simulink model "fsk4_rx"  (R2020b)
settings: Solver=VariableStepAuto  StartTime=0.0  StopTime=2/100e3  RelTol=1e-3
PreLoadFcn:
  | setup_receiver
InitFcn:
  | setup_receiver;
  | fs=100e3;
undefined symbols (not defined in the file): AXI4, Lite
libraries: xbsIndex_r4 x242, hdlsllib x16, commrandsrc3 x2, dsphdlxfrm x1
(part 1 of 2)
settings Model: Creator=s1553558  LastModifiedBy=s1553558

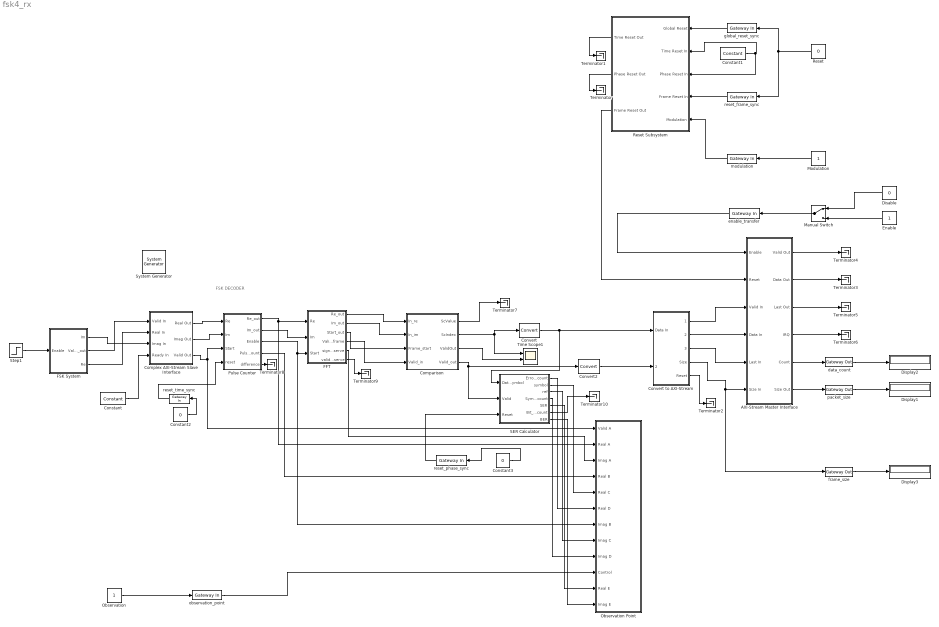
== system fsk4_rx ==
  note: FSK DECODER
  " System Generator" : xbsIndex_r4/ System Generator  Tag=genX  xilinxfamily=zynquplusRFSOC  part=xczu48dr  speed=-1-e  package=ffvg1517  synthesis_tool=Vivado  clock_wrapper=Clock Enables  directory=./netlist  proj_type=Vivado  Synth_file=Vivado Synthesis Defaults  Impl_file=Vivado Implementation Defaults  testbench=off  simulink_period=1/128e6  sysclk_period=(1/128e6)*1e9  dcm_input_clock_period=10  incr_netlist=off  trim_vbits=Everywhere in SubSystem  dbl_ovrd=According to Block Masks  core_generation=According to Block Masks  run_coregen=off  deprecated_control=off  eval_field=0  block_type=sysgen
  AXI-Stream Master Interface : Subsystem
  Comparison : Subsystem
  Complex AXI-Stream Slave Interface : Subsystem
  Constant : xbsIndex_r4/Constant  const=1.0  gui_display_data_type=Fixed-point  arith_type=Unsigned  n_bits=1  bin_pt=0  preci_type=Single  exp_width=8  frac_width=24  explicit_period=on  period=1/128e6  equ=P=C  opselect=C  inp2=PCIN>>17  opr=+  inp1=P  carry=CIN  dbl_ovrd=off  block_type=constant
  Constant1 : xbsIndex_r4/Constant  const=0  gui_display_data_type=Boolean  arith_type=Boolean  n_bits=16  bin_pt=14  preci_type=Single  exp_width=8  frac_width=24  explicit_period=on  period=1/128e6  equ=P=C  opselect=C  inp2=PCIN>>17  opr=+  inp1=P  carry=CIN  dbl_ovrd=off  block_type=constant
  Constant2 : Constant  Value=0
  Constant3 : Constant  Value=0
  Convert : xbsIndex_r4/Convert  gui_display_data_type=Fixed-point  arith_type=Unsigned  n_bits=8  bin_pt=0  float_type=Single  exp_bits=8  fraction_bits=24  quantization=Truncate  overflow=Wrap  en=off  latency=0  pipeline=off  dbl_ovrd=off  block_type=convert
  Convert to AXI-Stream : Subsystem
  Convert2 : xbsIndex_r4/Convert  gui_display_data_type=Boolean  arith_type=Boolean  n_bits=2  bin_pt=0  float_type=Single  exp_bits=8  fraction_bits=24  quantization=Truncate  overflow=Wrap  en=off  latency=0  pipeline=off  dbl_ovrd=off  block_type=convert
  Disable : Constant  Value=0  OutDataTypeStr=boolean  SampleTime=-1
  Display1 : Display
  Display2 : Display
  Display3 : Display
  Enable : Constant  OutDataTypeStr=boolean  SampleTime=-1
  FFT : Subsystem
  FSK System : Subsystem
  Manual Switch : ManualSwitch
  Modulation : Constant  OutDataTypeStr=boolean  SampleTime=-1
  Observation : Constant  OutDataTypeStr=uint32  SampleTime=-1
  Observation Point : Subsystem
  Pulse Counter : Subsystem
  Reset : Constant  Value=0  OutDataTypeStr=boolean  SampleTime=-1
  Reset Subsystem : Subsystem
  SER Calculator : Subsystem
  Step1 : Step  Time=32/128e6  SampleTime=32/128e6
  Terminator{,1..10} (11 alike) : Terminator
  Time Scope1 : Scope  NumInputPorts=2
  data_count : xbsIndex_r4/Gateway Out  inherit_from_input=on  hdl_port=on  rows=1  columns=1  UseAsDAC=off  DACChannel='1'  interface=AXI4-Lite  automatic_assignment=off  address_offset=32  intf_name=''  intf_description=''  timing_constraint=None  locs_specified=off  LOCs={}  io_standard={}  block_type=gatewayout
  enable_transfer : xbsIndex_r4/Gateway In  gui_display_data_type=Boolean  arith_type=Boolean  n_bits=16  bin_pt=14  preci_type=Single  exp_width=8  frac_width=24  rows=1  columns=1  quantization="Round  (unbiased: +/- Inf)"  overflow=Saturate  period=1/128e6  UseAsADC=off  ADCChannel='1'  interface=AXI4-Lite  automatic_assignment=off  address_offset=28  intf_name=''  intf_description=''  default_value=0  timing_constraint=None  locs_specified=off  LOCs={}  io_standard={}  inherit_from_input=off  hdl_port=on  dbl_ovrd=off  block_type=gatewayin
  frame_size : xbsIndex_r4/Gateway Out  inherit_from_input=on  hdl_port=on  rows=1  columns=1  UseAsDAC=off  DACChannel='1'  interface=AXI4-Lite  automatic_assignment=off  address_offset=16  intf_name=''  intf_description=''  timing_constraint=None  locs_specified=off  LOCs={}  io_standard={}  block_type=gatewayout
  global_reset_sync : xbsIndex_r4/Gateway In  gui_display_data_type=Boolean  arith_type=Boolean  n_bits=16  bin_pt=14  preci_type=Single  exp_width=8  frac_width=24  rows=1  columns=1  quantization="Round  (unbiased: +/- Inf)"  overflow=Saturate  period=1/4e6  UseAsADC=off  ADCChannel='1'  interface=AXI4-Lite  automatic_assignment=off  address_offset=56  intf_name=''  intf_description=''  default_value=1  timing_constraint=None  locs_specified=off  LOCs={}  io_standard={}  inherit_from_input=off  hdl_port=on  dbl_ovrd=off  block_type=gatewayin
  modulation : xbsIndex_r4/Gateway In  gui_display_data_type=Boolean  arith_type=Boolean  n_bits=16  bin_pt=14  preci_type=Single  exp_width=8  frac_width=24  rows=1  columns=1  quantization="Round  (unbiased: +/- Inf)"  overflow=Saturate  period=1/4e6  UseAsADC=off  ADCChannel='1'  interface=AXI4-Lite  automatic_assignment=off  address_offset=48  intf_name=''  intf_description=''  default_value=0  timing_constraint=None  locs_specified=off  LOCs={}  io_standard={}  inherit_from_input=off  hdl_port=on  dbl_ovrd=off  block_type=gatewayin
  observation_point : xbsIndex_r4/Gateway In  gui_display_data_type=Fixed-point  arith_type=Unsigned  n_bits=32  bin_pt=0  preci_type=Single  exp_width=8  frac_width=24  rows=1  columns=1  quantization="Round  (unbiased: +/- Inf)"  overflow=Saturate  period=1/128e6  UseAsADC=off  ADCChannel='1'  interface=AXI4-Lite  automatic_assignment=off  address_offset=36  intf_name=''  intf_description=''  default_value=0  timing_constraint=None  locs_specified=off  LOCs={}  io_standard={}  inherit_from_input=off  hdl_port=on  dbl_ovrd=off  block_type=gatewayin
  packet_size : xbsIndex_r4/Gateway Out  inherit_from_input=on  hdl_port=on  rows=1  columns=1  UseAsDAC=off  DACChannel='1'  interface=AXI4-Lite  automatic_assignment=off  address_offset=20  intf_name=''  intf_description=''  timing_constraint=None  locs_specified=off  LOCs={}  io_standard={}  block_type=gatewayout
  reset_frame_sync : xbsIndex_r4/Gateway In  gui_display_data_type=Boolean  arith_type=Boolean  n_bits=16  bin_pt=14  preci_type=Single  exp_width=8  frac_width=24  rows=1  columns=1  quantization="Round  (unbiased: +/- Inf)"  overflow=Saturate  period=1/4e6  UseAsADC=off  ADCChannel='1'  interface=AXI4-Lite  automatic_assignment=off  address_offset=8  intf_name=''  intf_description=''  default_value=1  timing_constraint=None  locs_specified=off  LOCs={}  io_standard={}  inherit_from_input=off  hdl_port=on  dbl_ovrd=off  block_type=gatewayin
  reset_phase_sync : xbsIndex_r4/Gateway In  gui_display_data_type=Boolean  arith_type=Boolean  n_bits=16  bin_pt=14  preci_type=Single  exp_width=8  frac_width=24  rows=1  columns=1  quantization="Round  (unbiased: +/- Inf)"  overflow=Saturate  period=1/4e6  UseAsADC=off  ADCChannel='1'  interface=AXI4-Lite  automatic_assignment=off  address_offset=4  intf_name=''  intf_description=''  default_value=1  timing_constraint=None  locs_specified=off  LOCs={}  io_standard={}  inherit_from_input=off  hdl_port=on  dbl_ovrd=off  block_type=gatewayin
  reset_time_sync : xbsIndex_r4/Gateway In  gui_display_data_type=Boolean  arith_type=Boolean  n_bits=16  bin_pt=14  preci_type=Single  exp_width=8  frac_width=24  rows=1  columns=1  quantization="Round  (unbiased: +/- Inf)"  overflow=Saturate  period=1/4e6  UseAsADC=off  ADCChannel='1'  interface=AXI4-Lite  automatic_assignment=off  address_offset=0  intf_name=''  intf_description=''  default_value=1  timing_constraint=None  locs_specified=off  LOCs={}  io_standard={}  inherit_from_input=off  hdl_port=on  dbl_ovrd=off  block_type=gatewayin
  wires:
  FSK System/3(Re) -> Complex AXI-Stream Slave Interface/2(Real In)
  FSK System/1(Im) -> Complex AXI-Stream Slave Interface/3(Imag In)
  FSK System/2(Valid_out) -> Complex AXI-Stream Slave Interface/1(Valid In)
  Step1/1 -> FSK System/1(Enable)
  Observation/1 -> observation_point/1
  Pulse Counter/3(Enable) -> Observation Point/7(Imag B), FFT/3(Start)
  FFT/2(Im_out) -> Comparison/2(In_im)
  FFT/1(Re_out) -> Comparison/1(In_re)
  Comparison/2(ScIndex) -> Time Scope1/1, Convert/1
  Pulse Counter/1(Re_out) -> Observation Point/2(Real A), FFT/1(Re)
  FFT/3(Start_out) -> Comparison/3(Frame_start)
  observation_point/1 -> Observation Point/10(Control)
  Pulse Counter/2(Im_out) -> FFT/2(Im)
  Constant1/1 -> Reset Subsystem/3(Phase Reset In), Reset Subsystem/2(Time Reset In)
  Modulation/1 -> modulation/1
  modulation/1 -> Reset Subsystem/5(Modulation)
  global_reset_sync/1 -> Reset Subsystem/1(Global Reset)
  reset_frame_sync/1 -> Reset Subsystem/4(Frame Reset In)
  Reset/1 -> global_reset_sync/1, reset_frame_sync/1
  Disable/1 -> Manual Switch/1
  enable_transfer/1 -> AXI-Stream Master Interface/1(Enable)
  Manual Switch/1 -> enable_transfer/1
  Enable/1 -> Manual Switch/2
  Reset Subsystem/3(Frame Reset Out) -> AXI-Stream Master Interface/2(Reset)
  Reset Subsystem/2(Phase Reset Out) -> Terminator/1
  Reset Subsystem/1(Time Reset Out) -> Terminator1/1
  Convert to AXI-Stream/1(Valid Out) -> AXI-Stream Master Interface/3(Valid In)
  Convert to AXI-Stream/2(Data Out) -> AXI-Stream Master Interface/4(Data In)
  Convert to AXI-Stream/3(Last Out) -> AXI-Stream Master Interface/5(Last In)
  Convert to AXI-Stream/5(Reset) -> Terminator2/1
  Convert to AXI-Stream/4(Size) -> frame_size/1, AXI-Stream Master Interface/6(Size In)
  AXI-Stream Master Interface/3(Last Out) -> Terminator5/1
  AXI-Stream Master Interface/4(IRQ) -> Terminator6/1
  AXI-Stream Master Interface/2(Data Out) -> Terminator3/1
  AXI-Stream Master Interface/1(Valid Out) -> Terminator4/1
  frame_size/1 -> Display3/1
  packet_size/1 -> Display1/1
  data_count/1 -> Display2/1
  AXI-Stream Master Interface/5(Count) -> data_count/1
  AXI-Stream Master Interface/6(Size Out) -> packet_size/1
  Complex AXI-Stream Slave Interface/2(Imag Out) -> Pulse Counter/2(Im)
  Complex AXI-Stream Slave Interface/1(Real Out) -> Pulse Counter/1(Re)
  Constant/1 -> Complex AXI-Stream Slave Interface/4(Ready In)
  Comparison/1(ScValue) -> Terminator7/1
  Complex AXI-Stream Slave Interface/3(Valid Out) -> Pulse Counter/3(Start), Observation Point/1(Valid A)
  FFT/4(Valid_frame) -> Comparison/4(Valid_in)
  Pulse Counter/4(Pulse Count) -> Observation Point/4(Real B)
  Comparison/4(Valid_out) -> Convert2/1, SER Calculator/2(Valid)
  Pulse Counter/5(difference) -> Terminator8/1
  reset_time_sync/1 -> Pulse Counter/4(reset)
  Constant2/1 -> reset_time_sync/1
  SER Calculator/2(symbol) -> Observation Point/5(Real C)
  SER Calculator/3(ref) -> Observation Point/8(Imag C)
  reset_phase_sync/1 -> SER Calculator/3(Reset)
  Constant3/1 -> reset_phase_sync/1
  Comparison/3(ValidOut) -> Time Scope1/2
  Convert/1 -> Convert to AXI-Stream/1(Data In), SER Calculator/1(Data_Symbol)
  Convert2/1 -> Convert to AXI-Stream/2(Valid In)
  FFT/5(signal_observe) -> Observation Point/3(Imag A)
  SER Calculator/4(Symbol_count) -> Observation Point/9(Imag D)
  FFT/6(valid_observe) -> Terminator9/1
  SER Calculator/7(BER) -> Observation Point/12(Imag E)
  SER Calculator/6(Bit_error_count) -> Terminator10/1
  SER Calculator/1(Error_count) -> Observation Point/6(Real D)
  SER Calculator/5(SER) -> Observation Point/11(Real E)

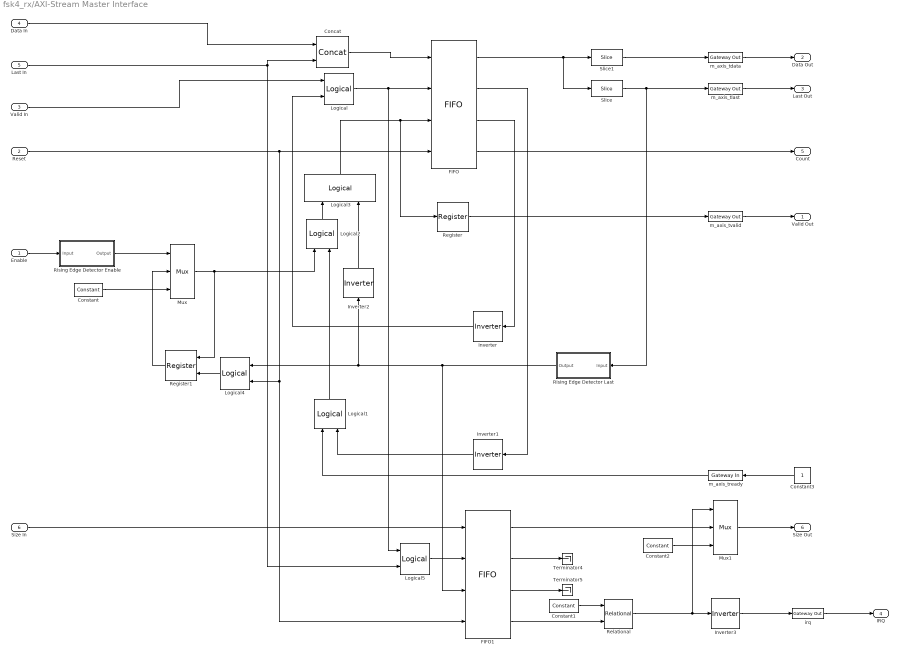
== system fsk4_rx/AXI-Stream Master Interface ==
  Enable : Inport
  Reset : Inport  Port=2
  Valid In : Inport  Port=3
  Data In : Inport  Port=4
  Last In : Inport  Port=5
  Size In : Inport  Port=6
  Concat : xbsIndex_r4/Concat  num_inputs=2  dbl_ovrd=off  block_type=concat
  Constant : xbsIndex_r4/Constant  const=1.0  gui_display_data_type=Boolean  arith_type=Boolean  n_bits=16  bin_pt=14  preci_type=Single  exp_width=8  frac_width=24  explicit_period=off  period=1  equ=P=C  opselect=C  inp2=PCIN>>17  opr=+  inp1=P  carry=CIN  dbl_ovrd=off  block_type=constant
  Constant1 : xbsIndex_r4/Constant  const=0  gui_display_data_type=Fixed-point  arith_type=Unsigned  n_bits=1  bin_pt=0  preci_type=Single  exp_width=8  frac_width=24  explicit_period=off  period=1  equ=P=C  opselect=C  inp2=PCIN>>17  opr=+  inp1=P  carry=CIN  dbl_ovrd=off  block_type=constant
  Constant2 : xbsIndex_r4/Constant  const=0  gui_display_data_type=Fixed-point  arith_type=Unsigned  n_bits=8  bin_pt=0  preci_type=Single  exp_width=8  frac_width=24  explicit_period=off  period=1  equ=P=C  opselect=C  inp2=PCIN>>17  opr=+  inp1=P  carry=CIN  dbl_ovrd=off  block_type=constant
  Constant3 : Constant  SampleTime=1/64e6
  FIFO : xbsIndex_r4/FIFO  mem_type=Block RAM  performance_options=Standard_FIFO  embedded_registers=off  depth=4K  percent_nbits=1  rst=on  rst_latency=2  en=off  use_dcount=on  use_percent_full_port=off  use_almost_empty=off  almost_empty_thresh=2  use_almost_full=off  use_rd_rst_busy=off  use_wr_rst_busy=off  almost_full_thresh=14  explicit_period=off  dbl_ovrd=off  simulation_type=fast_sim  block_type=fifo
  FIFO1 : xbsIndex_r4/FIFO  mem_type=Block RAM  performance_options=First_Word_Fall_Through  embedded_registers=off  depth=4K  percent_nbits=1  rst=on  rst_latency=2  en=off  use_dcount=on  use_percent_full_port=off  use_almost_empty=off  almost_empty_thresh=2  use_almost_full=off  use_rd_rst_busy=off  use_wr_rst_busy=off  almost_full_thresh=14  explicit_period=off  dbl_ovrd=off  simulation_type=fast_sim  block_type=fifo
  Inverter{,1..3} (4 alike) : xbsIndex_r4/Inverter  en=off  latency=0  dbl_ovrd=off  block_type=inv
  Logical{,1..3,5} (5 alike) : xbsIndex_r4/Logical  logical_function=AND  inputs=2  en=off  latency=0  precision=Full  arith_type=Unsigned  n_bits=16  bin_pt=0  align_bp=on  dbl_ovrd=off  block_type=logical
  Logical4 : xbsIndex_r4/Logical  logical_function=OR  inputs=2  en=off  latency=0  precision=Full  arith_type=Unsigned  n_bits=16  bin_pt=0  align_bp=on  dbl_ovrd=off  block_type=logical
  Mux : xbsIndex_r4/Mux  inputs=2  en=off  latency=0  precision=Full  arith_type=Unsigned  n_bits=16  bin_pt=14  quantization=Truncate  overflow=Wrap  dbl_ovrd=off  block_type=mux
  Mux1 : xbsIndex_r4/Mux  inputs=2  en=off  latency=0  precision=Full  arith_type=Unsigned  n_bits=16  bin_pt=14  quantization=Truncate  overflow=Wrap  dbl_ovrd=off  block_type=mux
  Register : xbsIndex_r4/Register  init=0  rst=off  en=off  dbl_ovrd=off  block_type=register
  Register1 : xbsIndex_r4/Register  init=0  rst=on  en=off  dbl_ovrd=off  block_type=register
  Relational : xbsIndex_r4/Relational  mode=a=b  op_type=Bool  en=off  latency=0  dbl_ovrd=off  block_type=relational
  Rising Edge Detector Enable : Subsystem
  Rising Edge Detector Last : Subsystem
  Slice : xbsIndex_r4/Slice  nbits=1  boolean_output=on  mode=Two Bit Locations  bit1=0  base1=LSB of Input  bit0=0  base0=LSB of Input  dbl_ovrd=off  block_type=slice
  Slice1 : xbsIndex_r4/Slice  nbits=1  boolean_output=off  mode=Two Bit Locations  bit1=8  base1=LSB of Input  bit0=1  base0=LSB of Input  dbl_ovrd=off  block_type=slice
  Terminator4 : Terminator
  Terminator5 : Terminator
  irq : xbsIndex_r4/Gateway Out  inherit_from_input=on  hdl_port=on  rows=1  columns=1  UseAsDAC=off  DACChannel='1'  interface=Interrupt  automatic_assignment=off  address_offset=36  intf_name=''  intf_description=''  timing_constraint=None  locs_specified=off  LOCs={}  io_standard={}  block_type=gatewayout
  m_axis_tdata : xbsIndex_r4/Gateway Out  inherit_from_input=on  hdl_port=on  rows=1  columns=1  UseAsDAC=off  DACChannel='1'  interface=None  automatic_assignment=on  address_offset=hex2dec('00')  intf_name=''  intf_description=''  timing_constraint=None  locs_specified=off  LOCs={}  io_standard={}  block_type=gatewayout
  m_axis_tlast : xbsIndex_r4/Gateway Out  inherit_from_input=on  hdl_port=on  rows=1  columns=1  UseAsDAC=off  DACChannel='1'  interface=None  automatic_assignment=on  address_offset=hex2dec('00')  intf_name=''  intf_description=''  timing_constraint=None  locs_specified=off  LOCs={}  io_standard={}  block_type=gatewayout
  m_axis_tready : xbsIndex_r4/Gateway In  gui_display_data_type=Boolean  arith_type=Boolean  n_bits=16  bin_pt=14  preci_type=Single  exp_width=8  frac_width=24  rows=1  columns=1  quantization="Round  (unbiased: +/- Inf)"  overflow=Saturate  period=1/128e6  UseAsADC=off  ADCChannel='1'  interface=None  automatic_assignment=on  address_offset=hex2dec('00')  intf_name=''  intf_description=''  default_value=0  timing_constraint=None  locs_specified=off  LOCs={}  io_standard={}  inherit_from_input=off  hdl_port=on  dbl_ovrd=off  block_type=gatewayin
  m_axis_tvalid : xbsIndex_r4/Gateway Out  inherit_from_input=on  hdl_port=on  rows=1  columns=1  UseAsDAC=off  DACChannel='1'  interface=None  automatic_assignment=on  address_offset=hex2dec('00')  intf_name=''  intf_description=''  timing_constraint=None  locs_specified=off  LOCs={}  io_standard={}  block_type=gatewayout
  Valid Out : Outport  VectorParamsAs1DForOutWhenUnconnected=off
  Data Out : Outport  Port=2  VectorParamsAs1DForOutWhenUnconnected=off
  Last Out : Outport  Port=3  VectorParamsAs1DForOutWhenUnconnected=off
  IRQ : Outport  Port=4  VectorParamsAs1DForOutWhenUnconnected=off
  Count : Outport  Port=5  VectorParamsAs1DForOutWhenUnconnected=off
  Size Out : Outport  Port=6  VectorParamsAs1DForOutWhenUnconnected=off
  wires:
  irq/1 -> IRQ/1
  Constant3/1 -> m_axis_tready/1
  Size In/1 -> FIFO1/1
  m_axis_tvalid/1 -> Valid Out/1
  m_axis_tlast/1 -> Last Out/1
  m_axis_tdata/1 -> Data Out/1
  FIFO/1 -> Slice1/1, Slice/1
  Logical/1 -> Logical5/1, FIFO/2
  FIFO/3 -> Inverter/1
  Inverter/1 -> Logical/2
  FIFO/2 -> Inverter1/1
  Inverter1/1 -> Logical1/2
  m_axis_tready/1 -> Logical1/1
  Concat/1 -> FIFO/1
  FIFO/4 -> Count/1
  Slice1/1 -> m_axis_tdata/1
  Register/1 -> m_axis_tvalid/1
  Logical1/1 -> Logical2/2
  Mux/1 -> Register1/1, Logical2/1
  Rising Edge Detector Enable/1(Output) -> Mux/1
  Register1/1 -> Mux/2
  Constant/1 -> Mux/3
  Enable/1 -> Rising Edge Detector Enable/1(Input)
  Slice/1 -> Rising Edge Detector Last/1(Input), m_axis_tlast/1
  Rising Edge Detector Last/1(Output) -> FIFO1/3, Inverter2/1, Logical4/1
  Logical3/1 -> FIFO/3, Register/1
  Logical2/1 -> Logical3/1
  Inverter2/1 -> Logical3/2
  Logical4/1 -> Register1/2
  FIFO1/2 -> Terminator4/1
  FIFO1/3 -> Terminator5/1
  FIFO1/4 -> Relational/2
  Logical5/1 -> FIFO1/2
  Constant1/1 -> Relational/1
  FIFO1/1 -> Mux1/2
  Mux1/1 -> Size Out/1
  Relational/1 -> Inverter3/1, Mux1/1
  Constant2/1 -> Mux1/3
  Inverter3/1 -> irq/1
  Data In/1 -> Concat/1
  Last In/1 -> Logical5/2, Concat/2
  Valid In/1 -> Logical/1
  Reset/1 -> FIFO/4, Logical4/2, FIFO1/4

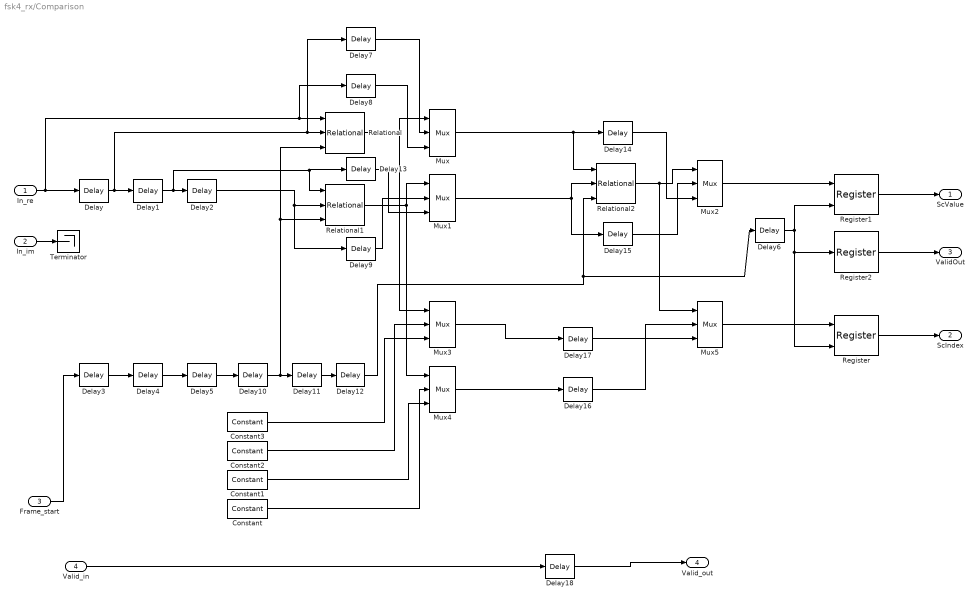
== system fsk4_rx/Comparison ==
  In_re : Inport
  In_im : Inport  Port=2
  Frame_start : Inport  Port=3
  Valid_in : Inport  Port=4
  Constant : xbsIndex_r4/Constant  const=0  gui_display_data_type=Fixed-point  arith_type=Unsigned  n_bits=16  bin_pt=14  preci_type=Single  exp_width=8  frac_width=24  explicit_period=on  period=1/128e6  equ=P=C  opselect=C  inp2=PCIN>>17  opr=+  inp1=P  carry=CIN  dbl_ovrd=off  block_type=constant
  Constant1 : xbsIndex_r4/Constant  const=1  gui_display_data_type=Fixed-point  arith_type=Unsigned  n_bits=16  bin_pt=14  preci_type=Single  exp_width=8  frac_width=24  explicit_period=on  period=1/128e6  equ=P=C  opselect=C  inp2=PCIN>>17  opr=+  inp1=P  carry=CIN  dbl_ovrd=off  block_type=constant
  Constant2 : xbsIndex_r4/Constant  const=2.0  gui_display_data_type=Fixed-point  arith_type=Unsigned  n_bits=16  bin_pt=14  preci_type=Single  exp_width=8  frac_width=24  explicit_period=on  period=1/128e6  equ=P=C  opselect=C  inp2=PCIN>>17  opr=+  inp1=P  carry=CIN  dbl_ovrd=off  block_type=constant
  Constant3 : xbsIndex_r4/Constant  const=3  gui_display_data_type=Fixed-point  arith_type=Unsigned  n_bits=16  bin_pt=14  preci_type=Single  exp_width=8  frac_width=24  explicit_period=on  period=1/128e6  equ=P=C  opselect=C  inp2=PCIN>>17  opr=+  inp1=P  carry=CIN  dbl_ovrd=off  block_type=constant
  Delay{,1..5,7..17} (17 alike) : xbsIndex_r4/Delay  rst=off  infoeditControl=Selection of Reset will increase slice count due to use of real FFs and instead of SRLs  en=off  latency=1  reg_retiming=off  dbl_ovrd=off  block_type=delay
  Delay18 : xbsIndex_r4/Delay  rst=off  infoeditControl=Selection of Reset will increase slice count due to use of real FFs and instead of SRLs  en=off  latency=8  reg_retiming=off  dbl_ovrd=off  block_type=delay
  Delay6 : xbsIndex_r4/Delay  rst=off  infoeditControl=Selection of Reset will increase slice count due to use of real FFs and instead of SRLs  en=off  latency=2  reg_retiming=off  dbl_ovrd=off  block_type=delay
  Mux{,1,3..4} (4 alike) : xbsIndex_r4/Mux  inputs=2  en=off  latency=1  precision=Full  arith_type=Unsigned  n_bits=16  bin_pt=14  quantization=Truncate  overflow=Wrap  dbl_ovrd=off  block_type=mux
  Mux2 : xbsIndex_r4/Mux  inputs=2  en=off  latency=1  precision=Full  arith_type="Signed  (2's comp)"  n_bits=16  bin_pt=14  quantization=Truncate  overflow=Wrap  dbl_ovrd=off  block_type=mux
  Mux5 : xbsIndex_r4/Mux  inputs=2  en=off  latency=1  precision=Full  arith_type="Signed  (2's comp)"  n_bits=16  bin_pt=14  quantization=Truncate  overflow=Wrap  dbl_ovrd=off  block_type=mux
  Register : xbsIndex_r4/Register  init=0  rst=off  en=on  dbl_ovrd=off  block_type=register
  Register1 : xbsIndex_r4/Register  init=0  rst=off  en=on  dbl_ovrd=off  block_type=register
  Register2 : xbsIndex_r4/Register  init=0  rst=off  en=off  dbl_ovrd=off  block_type=register
  Relational : xbsIndex_r4/Relational  mode=a>=b  op_type=Bool  en=on  latency=1  dbl_ovrd=off  block_type=relational
  Relational1 : xbsIndex_r4/Relational  mode=a>=b  op_type=Bool  en=on  latency=1  dbl_ovrd=off  block_type=relational
  Relational2 : xbsIndex_r4/Relational  mode=a>=b  op_type=Bool  en=on  latency=1  dbl_ovrd=off  block_type=relational
  Terminator : Terminator
  ScValue : Outport
  ScIndex : Outport  Port=2
  ValidOut : Outport  Port=3
  Valid_out : Outport  Port=4
  wires:
  Frame_start/1 -> Delay3/1
  Register1/1 -> ScValue/1
  In_re/1 -> Delay/1, Delay8/1, Relational/1
  Delay/1 -> Delay1/1, Delay7/1, Relational/2
  Delay2/1 -> Relational1/2, Delay9/1
  Relational/1 -> Mux/1, Mux3/1
  Mux/1 -> Relational2/1, Delay14/1
  Relational1/1 -> Mux4/1, Mux1/1
  Mux1/1 -> Delay15/1, Relational2/2
  Relational2/1 -> Mux5/1, Mux2/1
  Mux3/1 -> Delay17/1
  Mux4/1 -> Delay16/1
  Mux5/1 -> Register/1
  Register/1 -> ScIndex/1
  Delay10/1 -> Relational1/3, Relational/3, Delay11/1
  Delay3/1 -> Delay4/1
  Delay4/1 -> Delay5/1
  Delay5/1 -> Delay10/1
  Delay1/1 -> Relational1/1, Delay13/1, Delay2/1
  Delay11/1 -> Delay12/1
  Delay6/1 -> Register2/1, Register/2, Register1/2
  In_im/1 -> Terminator/1
  Delay7/1 -> Mux/2
  Delay8/1 -> Mux/3
  Delay9/1 -> Mux1/2
  Delay13/1 -> Mux1/3
  Delay14/1 -> Mux2/3
  Delay15/1 -> Mux2/2
  Mux2/1 -> Register1/1
  Delay12/1 -> Relational2/3, Delay6/1
  Constant3/1 -> Mux3/3
  Constant2/1 -> Mux3/2
  Constant/1 -> Mux4/2
  Constant1/1 -> Mux4/3
  Delay16/1 -> Mux5/2
  Delay17/1 -> Mux5/3
  Register2/1 -> ValidOut/1
  Valid_in/1 -> Delay18/1
  Delay18/1 -> Valid_out/1

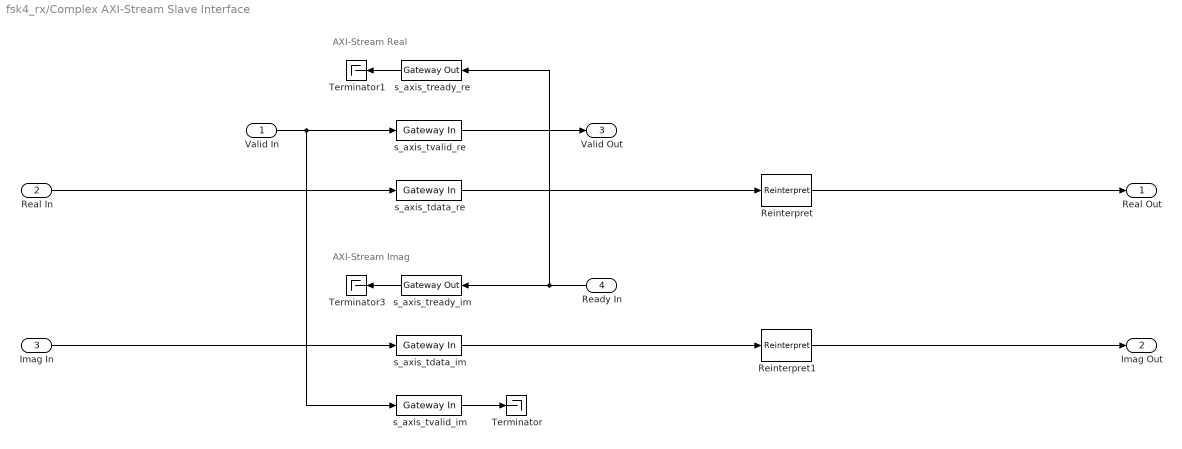
== system fsk4_rx/Complex AXI-Stream Slave Interface ==
  note: AXI-Stream Real
  note: AXI-Stream Imag
  Valid In : Inport
  Real In : Inport  Port=2
  Imag In : Inport  Port=3
  Ready In : Inport  Port=4
  Reinterpret : xbsIndex_r4/Reinterpret  force_arith_type=on  arith_type="Signed  (2's comp)"  force_bin_pt=on  bin_pt=14  block_type=reinterpret
  Reinterpret1 : xbsIndex_r4/Reinterpret  force_arith_type=on  arith_type="Signed  (2's comp)"  force_bin_pt=on  bin_pt=14  block_type=reinterpret
  Terminator : Terminator
  Terminator1 : Terminator
  Terminator3 : Terminator
  s_axis_tdata_im : xbsIndex_r4/Gateway In  gui_display_data_type=Fixed-point  arith_type=Unsigned  n_bits=16  bin_pt=0  preci_type=Double  exp_width=8  frac_width=24  rows=1  columns=1  quantization="Round  (unbiased: +/- Inf)"  overflow=Saturate  period=1/128e6  UseAsADC=off  ADCChannel='1'  interface=None  automatic_assignment=on  address_offset=hex2dec('00')  intf_name=''  intf_description=''  default_value=0  timing_constraint=None  locs_specified=off  LOCs={}  io_standard={}  inherit_from_input=off  hdl_port=on  dbl_ovrd=off  block_type=gatewayin
  s_axis_tdata_re : xbsIndex_r4/Gateway In  gui_display_data_type=Fixed-point  arith_type=Unsigned  n_bits=16  bin_pt=0  preci_type=Double  exp_width=8  frac_width=24  rows=1  columns=1  quantization="Round  (unbiased: +/- Inf)"  overflow=Saturate  period=1/128e6  UseAsADC=off  ADCChannel='1'  interface=None  automatic_assignment=on  address_offset=hex2dec('00')  intf_name=''  intf_description=''  default_value=0  timing_constraint=None  locs_specified=off  LOCs={}  io_standard={}  inherit_from_input=off  hdl_port=on  dbl_ovrd=off  block_type=gatewayin
  s_axis_tready_im : xbsIndex_r4/Gateway Out  inherit_from_input=off  hdl_port=on  rows=1  columns=1  UseAsDAC=off  DACChannel='1'  interface=None  automatic_assignment=on  address_offset=hex2dec('00')  intf_name=''  intf_description=''  timing_constraint=None  locs_specified=off  LOCs={}  io_standard={}  block_type=gatewayout
  s_axis_tready_re : xbsIndex_r4/Gateway Out  inherit_from_input=off  hdl_port=on  rows=1  columns=1  UseAsDAC=off  DACChannel='1'  interface=None  automatic_assignment=on  address_offset=hex2dec('00')  intf_name=''  intf_description=''  timing_constraint=None  locs_specified=off  LOCs={}  io_standard={}  block_type=gatewayout
  s_axis_tvalid_im : xbsIndex_r4/Gateway In  gui_display_data_type=Boolean  arith_type=Boolean  n_bits=16  bin_pt=14  preci_type=Single  exp_width=8  frac_width=24  rows=1  columns=1  quantization="Round  (unbiased: +/- Inf)"  overflow=Saturate  period=1/128e6  UseAsADC=off  ADCChannel='1'  interface=None  automatic_assignment=on  address_offset=hex2dec('00')  intf_name=''  intf_description=''  default_value=0  timing_constraint=None  locs_specified=off  LOCs={}  io_standard={}  inherit_from_input=off  hdl_port=on  dbl_ovrd=off  block_type=gatewayin
  s_axis_tvalid_re : xbsIndex_r4/Gateway In  gui_display_data_type=Boolean  arith_type=Boolean  n_bits=32  bin_pt=0  preci_type=Single  exp_width=8  frac_width=24  rows=1  columns=1  quantization="Round  (unbiased: +/- Inf)"  overflow=Saturate  period=1/128e6  UseAsADC=off  ADCChannel='1'  interface=None  automatic_assignment=on  address_offset=hex2dec('00')  intf_name=''  intf_description=''  default_value=0  timing_constraint=None  locs_specified=off  LOCs={}  io_standard={}  inherit_from_input=off  hdl_port=on  dbl_ovrd=off  block_type=gatewayin
  Real Out : Outport  VectorParamsAs1DForOutWhenUnconnected=off
  Imag Out : Outport  Port=2  VectorParamsAs1DForOutWhenUnconnected=off
  Valid Out : Outport  Port=3  VectorParamsAs1DForOutWhenUnconnected=off
  wires:
  s_axis_tready_re/1 -> Terminator1/1
  Valid In/1 -> s_axis_tvalid_re/1, s_axis_tvalid_im/1
  Ready In/1 -> s_axis_tready_im/1, s_axis_tready_re/1
  s_axis_tvalid_re/1 -> Valid Out/1
  s_axis_tvalid_im/1 -> Terminator/1
  s_axis_tready_im/1 -> Terminator3/1
  Imag In/1 -> s_axis_tdata_im/1
  Real In/1 -> s_axis_tdata_re/1
  s_axis_tdata_re/1 -> Reinterpret/1
  Reinterpret1/1 -> Imag Out/1
  s_axis_tdata_im/1 -> Reinterpret1/1
  Reinterpret/1 -> Real Out/1

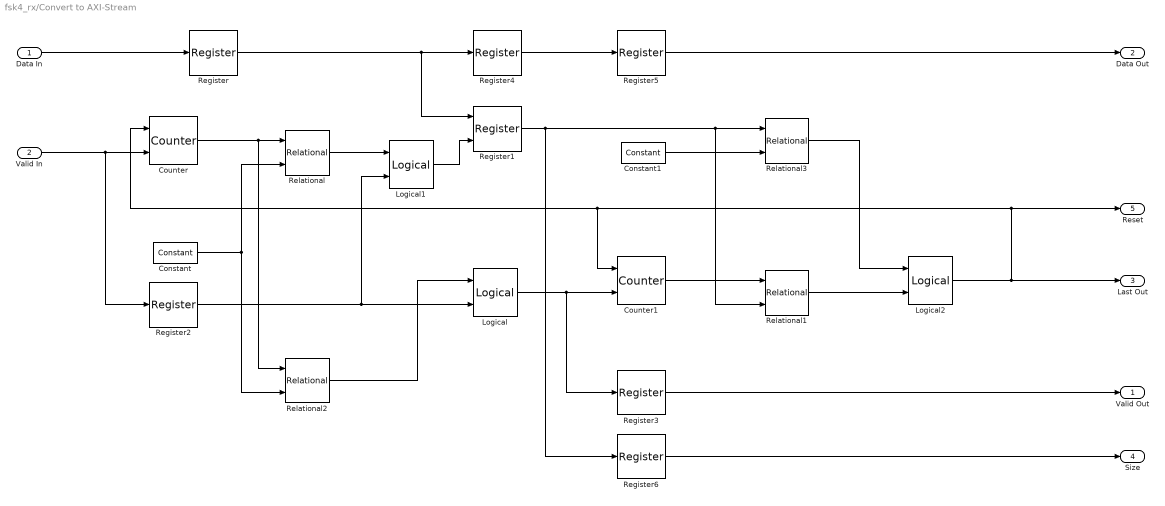
== system fsk4_rx/Convert to AXI-Stream ==
  Data In : Inport
  Valid In : Inport  Port=2
  Constant : xbsIndex_r4/Constant  const=1.0  gui_display_data_type=Fixed-point  arith_type=Unsigned  n_bits=1  bin_pt=0  preci_type=Single  exp_width=8  frac_width=24  explicit_period=off  period=1  equ=P=C  opselect=C  inp2=PCIN>>17  opr=+  inp1=P  carry=CIN  dbl_ovrd=off  block_type=constant
  Constant1 : xbsIndex_r4/Constant  const=0  gui_display_data_type=Fixed-point  arith_type=Unsigned  n_bits=1  bin_pt=0  preci_type=Single  exp_width=8  frac_width=24  explicit_period=off  period=1  equ=P=C  opselect=C  inp2=PCIN>>17  opr=+  inp1=P  carry=CIN  dbl_ovrd=off  block_type=constant
  Counter : xbsIndex_r4/Counter  cnt_type=Free Running  cnt_to=Inf  operation=Up  start_count=0  cnt_by_val=1  arith_type=Unsigned  n_bits=32  bin_pt=0  load_pin=off  rst=on  en=on  explicit_period=off  period=1  use_behavioral_HDL=off  implementation=Fabric  dbl_ovrd=off  block_type=counter
  Counter1 : xbsIndex_r4/Counter  cnt_type=Free Running  cnt_to=Inf  operation=Up  start_count=0  cnt_by_val=1  arith_type=Unsigned  n_bits=32  bin_pt=0  load_pin=off  rst=on  en=on  explicit_period=off  period=1  use_behavioral_HDL=off  implementation=Fabric  dbl_ovrd=off  block_type=counter
  Logical : xbsIndex_r4/Logical  logical_function=AND  inputs=2  en=off  latency=1  precision=Full  arith_type=Unsigned  n_bits=16  bin_pt=0  align_bp=on  dbl_ovrd=off  block_type=logical
  Logical1 : xbsIndex_r4/Logical  logical_function=AND  inputs=2  en=off  latency=0  precision=Full  arith_type=Unsigned  n_bits=16  bin_pt=0  align_bp=on  dbl_ovrd=off  block_type=logical
  Logical2 : xbsIndex_r4/Logical  logical_function=AND  inputs=2  en=off  latency=0  precision=Full  arith_type=Unsigned  n_bits=16  bin_pt=0  align_bp=on  dbl_ovrd=off  block_type=logical
  Register{,2..6} (6 alike) : xbsIndex_r4/Register  init=0  rst=off  en=off  dbl_ovrd=off  block_type=register
  Register1 : xbsIndex_r4/Register  init=0  rst=off  en=on  dbl_ovrd=off  block_type=register
  Relational : xbsIndex_r4/Relational  mode=a=b  op_type=Bool  en=off  latency=0  dbl_ovrd=off  block_type=relational
  Relational1 : xbsIndex_r4/Relational  mode=a>=b  op_type=Bool  en=off  latency=0  dbl_ovrd=off  block_type=relational
  Relational2 : xbsIndex_r4/Relational  mode=a>b  op_type=Bool  en=off  latency=0  dbl_ovrd=off  block_type=relational
  Relational3 : xbsIndex_r4/Relational  mode=a!=b  op_type=Bool  en=off  latency=0  dbl_ovrd=off  block_type=relational
  Valid Out : Outport  VectorParamsAs1DForOutWhenUnconnected=off
  Data Out : Outport  Port=2  VectorParamsAs1DForOutWhenUnconnected=off
  Last Out : Outport  Port=3  VectorParamsAs1DForOutWhenUnconnected=off
  Size : Outport  Port=4  VectorParamsAs1DForOutWhenUnconnected=off
  Reset : Outport  Port=5  VectorParamsAs1DForOutWhenUnconnected=off
  wires:
  Valid In/1 -> Register2/1, Counter/2
  Counter/1 -> Relational2/1, Relational/1
  Data In/1 -> Register/1
  Register/1 -> Register4/1, Register1/1
  Logical/1 -> Register3/1, Counter1/2
  Counter1/1 -> Relational1/1
  Register1/1 -> Register6/1, Relational3/1, Relational1/2
  Register2/1 -> Logical1/2, Logical/2
  Register3/1 -> Valid Out/1
  Register4/1 -> Register5/1
  Register5/1 -> Data Out/1
  Constant/1 -> Relational/2, Relational2/2
  Relational2/1 -> Logical/1
  Relational/1 -> Logical1/1
  Logical1/1 -> Register1/2
  Constant1/1 -> Relational3/2
  Relational3/1 -> Logical2/1
  Relational1/1 -> Logical2/2
  Logical2/1 -> Counter/1, Counter1/1, Reset/1, Last Out/1
  Register6/1 -> Size/1

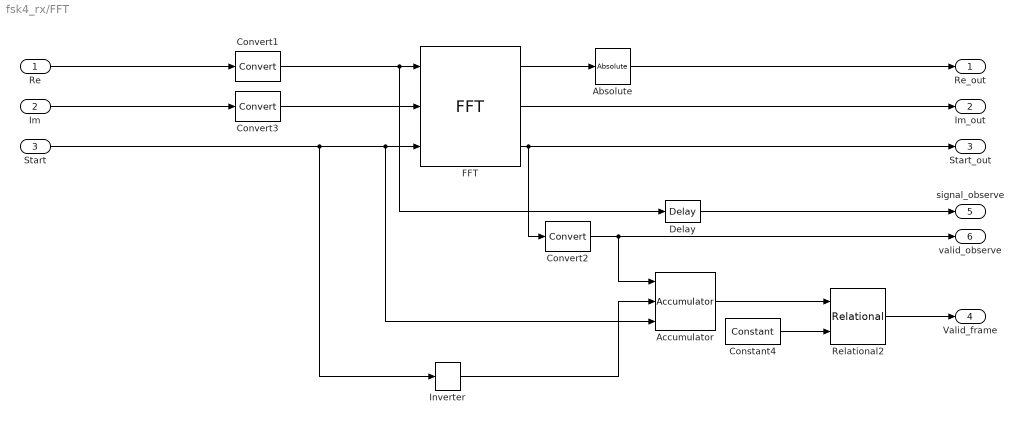
== system fsk4_rx/FFT ==
  Re : Inport
  Im : Inport  Port=2
  Start : Inport  Port=3
  Absolute : xbsIndex_r4/Absolute  precision=Full  arith_type=Unsigned  n_bits=16  bin_pt=14  quantization=Truncate  overflow=Wrap  en=off  latency=0  dbl_ovrd=off  block_type=abs
  Accumulator : xbsIndex_r4/Accumulator  operation=Add  n_bits=54  overflow=Wrap  scale=1  rst=on  hasbypass=off  infoeditControl=reset for floating point data type must be asserted for a minimum of 2 cycles  en=on  latency=0  msb_inp=100  msb=100  lsb=-100  use_behavioral_HDL=on  implementation=Fabric  dbl_ovrd=off  block_type=accum
  Constant4 : xbsIndex_r4/Constant  const=0.1  gui_display_data_type=Fixed-point  arith_type=Unsigned  n_bits=16  bin_pt=14  preci_type=Single  exp_width=8  frac_width=24  explicit_period=on  period=1/128e6  equ=P=C  opselect=C  inp2=PCIN>>17  opr=+  inp1=P  carry=CIN  dbl_ovrd=off  block_type=constant
  Convert1 : xbsIndex_r4/Convert  gui_display_data_type=Fixed-point  arith_type="Signed  (2's comp)"  n_bits=32  bin_pt=16  float_type=Single  exp_bits=8  fraction_bits=24  quantization=Truncate  overflow=Wrap  en=off  latency=0  pipeline=off  dbl_ovrd=off  block_type=convert
  Convert2 : xbsIndex_r4/Convert  gui_display_data_type=Fixed-point  arith_type=Unsigned  n_bits=16  bin_pt=14  float_type=Single  exp_bits=8  fraction_bits=24  quantization=Truncate  overflow=Wrap  en=off  latency=0  pipeline=off  dbl_ovrd=off  block_type=convert
  Convert3 : xbsIndex_r4/Convert  gui_display_data_type=Fixed-point  arith_type="Signed  (2's comp)"  n_bits=32  bin_pt=16  float_type=Single  exp_bits=8  fraction_bits=24  quantization=Truncate  overflow=Wrap  en=off  latency=0  pipeline=off  dbl_ovrd=off  block_type=convert
  Delay : xbsIndex_r4/Delay  rst=off  infoeditControl=Selection of Reset will increase slice count due to use of real FFs and instead of SRLs  en=off  latency=164  reg_retiming=off  dbl_ovrd=off  block_type=delay
  FFT : xbsIndex_r4/FFT  infoeditControl=Hardware notes: This block implements a burst IO radix-2 architecture if the <b><i>Optimize for</i></b> parameter is selected as <b><i>Resources</i></b>, and the input sample period is 8 times slower than the system sample period; otherwise a pipeline streaming architecture will be used.  transform_length=32  scale_result_by_fft_length=off  bit_reversed_order=on  optimizegoal=Resources  start_frame=on  simulation_type=fast_sim  simulation_model=sysgen:ForwardFFT_Macro  latency=1  block_type=xfft_forward
  Inverter : xbsIndex_r4/Inverter  en=off  latency=0  dbl_ovrd=off  block_type=inv
  Relational2 : xbsIndex_r4/Relational  mode=a>b  op_type=Ufix  en=off  latency=0  dbl_ovrd=off  block_type=relational
  Re_out : Outport
  Im_out : Outport  Port=2
  Start_out : Outport  Port=3
  Valid_frame : Outport  Port=4
  signal_observe : Outport  Port=5
  valid_observe : Outport  Port=6
  wires:
  Re/1 -> Convert1/1
  FFT/1 -> Absolute/1
  Im/1 -> Convert3/1
  Convert2/1 -> Accumulator/1, valid_observe/1
  Accumulator/1 -> Relational2/1
  Inverter/1 -> Accumulator/2
  Relational2/1 -> Valid_frame/1
  Constant4/1 -> Relational2/2
  FFT/3 -> Start_out/1, Convert2/1
  FFT/2 -> Im_out/1
  Absolute/1 -> Re_out/1
  Start/1 -> Inverter/1, Accumulator/3, FFT/3
  Convert1/1 -> Delay/1, FFT/1
  Convert3/1 -> FFT/2
  Delay/1 -> signal_observe/1

== system fsk4_rx/FSK System ==
  Enable : Inport
  Bernoulli Binary Generator : commrandsrc3/Bernoulli Binary Generator  ProbabilityOfZero=0.5  SeedSource=Parameter  Seed=53  SampleTime=32/128e6  SamplesPerFrame=1  OutputDataType=boolean  SimulateUsing=Interpreted execution
  Bernoulli Binary Generator1 : commrandsrc3/Bernoulli Binary Generator  ProbabilityOfZero=0.5  SeedSource=Parameter  Seed=1  SampleTime=32/128e6  SamplesPerFrame=1  OutputDataType=boolean  SimulateUsing=Interpreted execution
  Cast1 : DataTypeConversion  OutDataTypeStr=double
  Complex to Real-Imag : ComplexToRealImag
  FSK Frame Generator : Subsystem
  Multiport Switch1 : MultiPortSwitch  DataPortOrder=Zero-based contiguous  Inputs=2  zeroidx=on
  Real-Imag to Complex : RealImagToComplex
  Square Wave Generator : SignalGenerator  WaveForm=square  Amplitude=2  Frequency=12.8e6
  Im : Outport  VectorParamsAs1DForOutWhenUnconnected=off
  Valid_out : Outport  Port=2  VectorParamsAs1DForOutWhenUnconnected=off
  Re : Outport  Port=3  VectorParamsAs1DForOutWhenUnconnected=off
  wires:
  Enable/1 -> FSK Frame Generator/2(modulation), FSK Frame Generator/1(tx_data)
  Bernoulli Binary Generator1/1 -> FSK Frame Generator/3(s_re_tdata)
  Bernoulli Binary Generator/1 -> FSK Frame Generator/4(s_im_tdata1)
  FSK Frame Generator/2(m_im_tdata) -> Real-Imag to Complex/2
  FSK Frame Generator/1(m_re_tdata) -> Real-Imag to Complex/1
  Real-Imag to Complex/1 -> Complex to Real-Imag/1
  Square Wave Generator/1 -> Multiport Switch1/2
  Complex to Real-Imag/1 -> Multiport Switch1/3
  Cast1/1 -> Multiport Switch1/1
  Complex to Real-Imag/2 -> Im/1
  FSK Frame Generator/3(m_tvalid) -> Valid_out/1, Cast1/1
  Multiport Switch1/1 -> Re/1

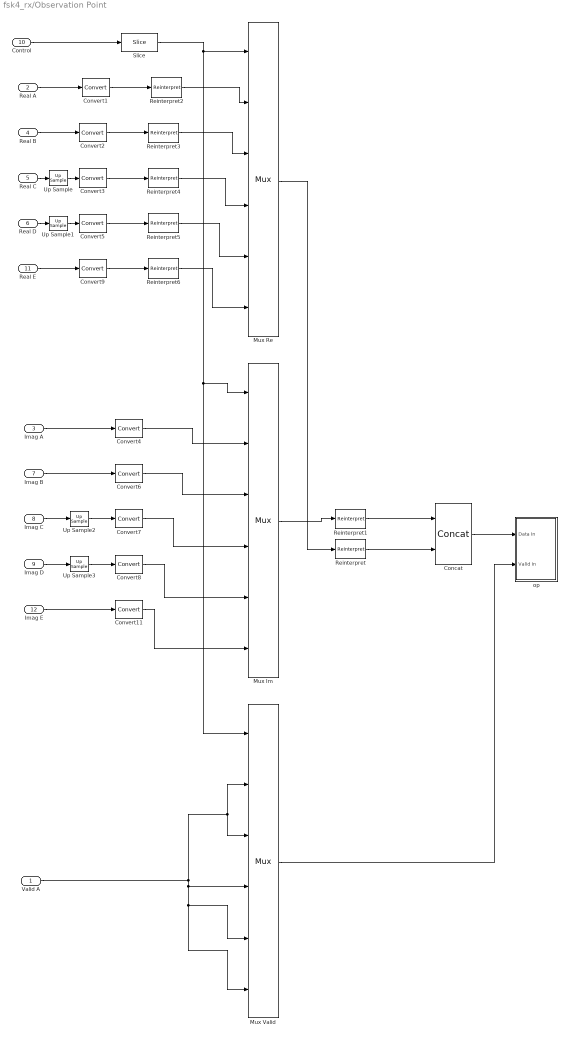
== system fsk4_rx/Observation Point ==
  Valid A : Inport
  Real A : Inport  Port=2
  Imag A : Inport  Port=3
  Real B : Inport  Port=4
  Real C : Inport  Port=5
  Real D : Inport  Port=6
  Imag B : Inport  Port=7
  Imag C : Inport  Port=8
  Imag D : Inport  Port=9
  Control : Inport  Port=10
  Real E : Inport  Port=11
  Imag E : Inport  Port=12
  Concat : xbsIndex_r4/Concat  num_inputs=2  dbl_ovrd=off  block_type=concat
  Convert{1..9,11} (10 alike) : xbsIndex_r4/Convert  gui_display_data_type=Fixed-point  arith_type="Signed  (2's comp)"  n_bits=16  bin_pt=5  float_type=Single  exp_bits=8  fraction_bits=24  quantization=Truncate  overflow=Wrap  en=off  latency=0  pipeline=off  dbl_ovrd=off  block_type=convert
  Mux Im : xbsIndex_r4/Mux  inputs=5  en=off  latency=1  precision=Full  arith_type=Unsigned  n_bits=16  bin_pt=14  quantization=Truncate  overflow=Wrap  dbl_ovrd=off  block_type=mux
  Mux Re : xbsIndex_r4/Mux  inputs=5  en=off  latency=1  precision=Full  arith_type=Unsigned  n_bits=16  bin_pt=14  quantization=Truncate  overflow=Wrap  dbl_ovrd=off  block_type=mux
  Mux Valid : xbsIndex_r4/Mux  inputs=5  en=off  latency=1  precision=Full  arith_type=Unsigned  n_bits=16  bin_pt=14  quantization=Truncate  overflow=Wrap  dbl_ovrd=off  block_type=mux
  Reinterpret{,1..6} (7 alike) : xbsIndex_r4/Reinterpret  force_arith_type=on  arith_type=Unsigned  force_bin_pt=on  bin_pt=0  block_type=reinterpret
  Slice : xbsIndex_r4/Slice  nbits=1  boolean_output=off  mode=Two Bit Locations  bit1=2  base1=LSB of Input  bit0=0  base0=LSB of Input  dbl_ovrd=off  block_type=slice
  Up Sample{,1..3} (4 alike) : xbsIndex_r4/Up Sample  sample_ratio=32  copy_samples=on  en=off  latency=0  dbl_ovrd=off  block_type=usamp
  op : Subsystem
  wires:
  Control/1 -> Slice/1
  Concat/1 -> op/1(Data In)
  Mux Re/1 -> Reinterpret/1
  Mux Valid/1 -> op/2(Valid In)
  Imag A/1 -> Convert4/1
  Mux Im/1 -> Reinterpret1/1
  Slice/1 -> Mux Valid/1, Mux Im/1, Mux Re/1
  Reinterpret1/1 -> Concat/1
  Reinterpret/1 -> Concat/2
  Convert1/1 -> Reinterpret2/1
  Convert4/1 -> Mux Im/2
  Valid A/1 -> Mux Valid/4, Mux Valid/6, Mux Valid/5, Mux Valid/2, Mux Valid/3
  Real A/1 -> Convert1/1
  Real B/1 -> Convert2/1
  Convert3/1 -> Reinterpret4/1
  Imag B/1 -> Convert6/1
  Convert6/1 -> Mux Im/3
  Convert7/1 -> Mux Im/4
  Convert8/1 -> Mux Im/5
  Reinterpret2/1 -> Mux Re/2
  Reinterpret3/1 -> Mux Re/3
  Reinterpret4/1 -> Mux Re/4
  Reinterpret5/1 -> Mux Re/5
  Convert2/1 -> Reinterpret3/1
  Real C/1 -> Up Sample/1
  Real D/1 -> Up Sample1/1
  Imag C/1 -> Up Sample2/1
  Imag D/1 -> Up Sample3/1
  Convert5/1 -> Reinterpret5/1
  Convert9/1 -> Reinterpret6/1
  Real E/1 -> Convert9/1
  Reinterpret6/1 -> Mux Re/6
  Imag E/1 -> Convert11/1
  Convert11/1 -> Mux Im/6
  Up Sample/1 -> Convert3/1
  Up Sample1/1 -> Convert5/1
  Up Sample2/1 -> Convert7/1
  Up Sample3/1 -> Convert8/1
